simulink model "tp095221"  (Simulink 5.1)
settings: Solver=ode5  SolverMode=SingleTasking  StartTime=0.0  StopTime=3  FixedStep=1/fc  RelTol=1e-3  AbsTol=1e-6
values from neighbouring files (symbols this model uses):
  A1 = 1/3    (= 0.333333333333)    [ADC.m]
  A2 = 1/4    (= 0.25)    [ADC.m]
  A3 = 1/5    (= 0.2)    [ADC.m]
  b = 4    [ADC.m]
  den_d = den_d{1,1}    [ADC.m]
  f1 = -fmax:df:fmax-df    [ADC.m]
  f2 = -fmax*N:df:fmax*N-df    [ADC.m]
  f3 = -fmax:df:fmax-df    [ADC.m]
  fs = 30    [ADC.m]
  k = 2    [ADC.m]
  N = 30    [ADC.m]
  num_d = num_d{1,1}    [ADC.m]
settings Model: LastModifiedBy=Sommer  SaveFormat=Matrix

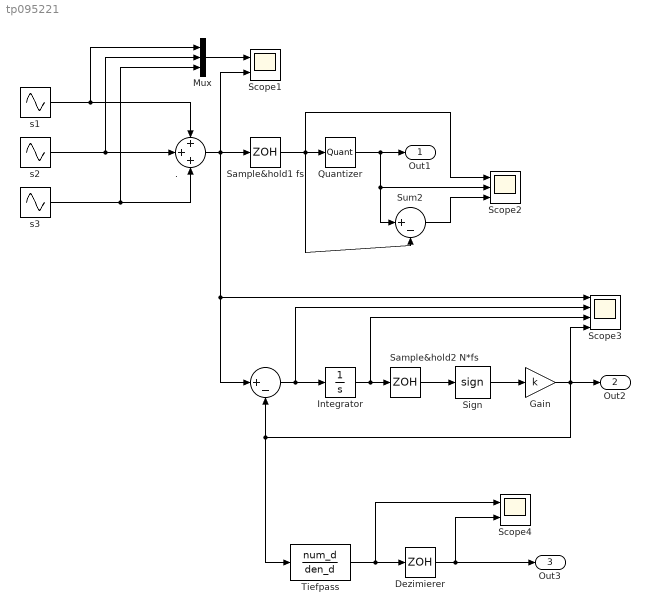
== system tp095221 ==
  " " : Sum  Inputs=|+-  SaturateOnIntegerOverflow=on
  . : Sum  Inputs=+++  SaturateOnIntegerOverflow=on
  Dezimierer : ZeroOrderHold  SampleTime=1/fs
  Gain : Gain  Gain=k  SaturateOnIntegerOverflow=on
  Integrator : Integrator  ExternalReset=none  InitialConditionSource=internal  InitialCondition=0  LimitOutput=off  UpperSaturationLimit=inf  LowerSaturationLimit=-inf  ShowSaturationPort=off  ShowStatePort=off  AbsoluteTolerance=auto
  Mux : Mux  Inputs=3
  Quantizer : Quantizer  QuantizationInterval=1/2^(b-1)
  Sample&hold1 fs : ZeroOrderHold  SampleTime=1/fs
  Sample&hold2 N*fs : ZeroOrderHold  SampleTime=1/(N*fs)
  Scope1 : Scope  NumInputPorts=2
      settings: TickLabels=on  TimeRange=3  YMin=-0.4~-0.8  YMax=0.4~0.8  SaveToWorkspace=off  SaveName=ScopeData  DataFormat=Matrix
  Scope2 : Scope  NumInputPorts=3
      settings: TickLabels=on  TimeRange=3  YMin=-0.8~-0.8~-0.06  YMax=0.8~0.8~0.06  SaveToWorkspace=off
  Scope3 : Scope  NumInputPorts=4
      settings: TickLabels=on  TimeRange=3  YMin=-1~-4~-0.005~-4  YMax=1~4~0.005~4  SaveToWorkspace=off  SaveName=ScopeData  DataFormat=Matrix
  Scope4 : Scope  NumInputPorts=2
      settings: TickLabels=on  TimeRange=3  YMin=-1~-1  YMax=1~1  SaveToWorkspace=off  SaveName=ScopeData  DataFormat=Matrix
  Sign : Signum
  Sum2 : Sum  Inputs=|+-  SaturateOnIntegerOverflow=on
  Tiefpass : DiscreteTransferFcn  Numerator=num_d  Denominator=den_d  SampleTime=-1
  s1 : Sin  Amplitude=A1  Frequency=2*pi*f1  Phase=0  SampleTime=0
  s2 : Sin  Amplitude=A2  Frequency=2*pi*f2  Phase=0  SampleTime=0
  s3 : Sin  Amplitude=A3  Frequency=2*pi*f3  Phase=0  SampleTime=0
  Out1 : Outport  Port=1
  Out2 : Outport  Port=2
  Out3 : Outport  Port=3
  wires:
  s1/1 -> Mux/1, ./1
  Quantizer/1 -> Out1/1, Sum2/1, Scope2/2
  Gain/1 -> Out2/1, " "/2, Tiefpass/1, Scope3/4
  " "/1 -> Integrator/1, Scope3/2
  Sum2/1 -> Scope2/3
  s3/1 -> Mux/3, ./3
  Integrator/1 -> Sample&hold2 N*fs/1, Scope3/3
  Sample&hold2 N*fs/1 -> Sign/1
  Sign/1 -> Gain/1
  Sample&hold1 fs/1 -> Sum2/2, Quantizer/1, Scope2/1
  Tiefpass/1 -> Dezimierer/1, Scope4/1
  Dezimierer/1 -> Out3/1, Scope4/2
  s2/1 -> ./2, Mux/2
  Mux/1 -> Scope1/1
  ./1 -> Sample&hold1 fs/1, Scope1/2, " "/1, Scope3/1
